simulink model "flatball_hummel_mdl_validation_IC"  (R2021b)
settings: Solver=ode1be  StartTime=0.0  StopTime=30  FixedStep=0.001  MaxStep=0.01  MinStep=0.01  RelTol=1e-3
values from neighbouring files (symbols this model uses):
  amb = evalin( 'base', 'amb')    [flatball_6dof_eqom.m]
  disc = evalin( 'base', 'disc')    [flatball_6dof_eqom.m]    (also in flatball_6dof_init.m = struct; flatball_init_disc_params.m = struct)
  k_launch_F_t_release = 0.60    (= 0.6)    [flatball_6dof_hucker_init.m]
  k_launch_Fx_kd = 2e-2    (= 0.02)    [flatball_6dof_hucker_init.m]
  k_launch_Fx_ki = 15    [flatball_6dof_hucker_init.m]
  k_launch_Fx_kp = 7.5    [flatball_6dof_hucker_init.m]
  k_launch_Fx_sat_hi = 150    [flatball_6dof_hucker_init.m]
  k_launch_Fx_sat_lo = -150    [flatball_6dof_hucker_init.m]
  k_launch_Fx_t_launch_begin = 0.50    (= 0.5)    [flatball_6dof_hucker_init.m]
  k_launch_Fx_t_launch_end = k_launch_F_t_release    (= 0.6)    [flatball_6dof_hucker_init.m]
  k_launch_Fx_tau = 1e-2    (= 0.01)    [flatball_6dof_hucker_init.m]
  k_launch_Fy_kd = k_launch_Fx_kd    (= 0.02)    [flatball_6dof_hucker_init.m]
  k_launch_Fy_ki = k_launch_Fx_ki    (= 15)    [flatball_6dof_hucker_init.m]
  k_launch_Fy_kp = k_launch_Fx_kp    (= 7.5)    [flatball_6dof_hucker_init.m]
  k_launch_Fy_sat_hi = k_launch_Fx_sat_hi    (= 150)    [flatball_6dof_hucker_init.m]
  k_launch_Fy_sat_lo = k_launch_Fx_sat_lo    (= -150)    [flatball_6dof_hucker_init.m]
  k_launch_Fy_t_launch_begin = 0.50    (= 0.5)    [flatball_6dof_hucker_init.m]
  k_launch_Fy_t_launch_end = k_launch_F_t_release    (= 0.6)    [flatball_6dof_hucker_init.m]
  k_launch_Fy_tau = 1e-2    (= 0.01)    [flatball_6dof_hucker_init.m]
  k_launch_Fz_kd = 2.5    [flatball_6dof_hucker_init.m]
  k_launch_Fz_ki = 50    [flatball_6dof_hucker_init.m]
  k_launch_Fz_kp = 20    [flatball_6dof_hucker_init.m]
  k_launch_Fz_sat_hi = 25    [flatball_6dof_hucker_init.m]
  k_launch_Fz_sat_lo = -25    [flatball_6dof_hucker_init.m]
  k_launch_Fz_t_launch_begin = 0.10    (= 0.1)    [flatball_6dof_hucker_init.m]
  k_launch_Fz_t_launch_end = k_launch_F_t_release    (= 0.6)    [flatball_6dof_hucker_init.m]
  k_launch_Fz_tau = 1e-2    (= 0.01)    [flatball_6dof_hucker_init.m]
  k_launch_M_t_release = 0.60    (= 0.6)    [flatball_6dof_hucker_init.m]
  k_launch_Mx_kd = 0.125    [flatball_6dof_hucker_init.m]
  k_launch_Mx_ki = 1.125    [flatball_6dof_hucker_init.m]
  k_launch_Mx_kp = 3.5    [flatball_6dof_hucker_init.m]
  k_launch_Mx_sat_hi = 2.5    [flatball_6dof_hucker_init.m]
  k_launch_Mx_sat_lo = -2.5    [flatball_6dof_hucker_init.m]
  k_launch_Mx_t_launch_begin = 0.30    (= 0.3)    [flatball_6dof_hucker_init.m]
  k_launch_Mx_t_launch_end = k_launch_M_t_release    (= 0.6)    [flatball_6dof_hucker_init.m]
  k_launch_Mx_tau = 1e-2    (= 0.01)    [flatball_6dof_hucker_init.m]
  k_launch_My_kd = 0.1125    [flatball_6dof_hucker_init.m]
  k_launch_My_ki = 5.5    [flatball_6dof_hucker_init.m]
  k_launch_My_kp = 4.25    [flatball_6dof_hucker_init.m]
  k_launch_My_sat_hi = 2.5    [flatball_6dof_hucker_init.m]
  k_launch_My_sat_lo = -2.5    [flatball_6dof_hucker_init.m]
  k_launch_My_t_launch_begin = 0.40    (= 0.4)    [flatball_6dof_hucker_init.m]
  k_launch_My_t_launch_end = k_launch_M_t_release    (= 0.6)    [flatball_6dof_hucker_init.m]
  k_launch_My_tau = 1e-2    (= 0.01)    [flatball_6dof_hucker_init.m]
  k_launch_Mz_kd = 1e-8    (= 1e-08)    [flatball_6dof_hucker_init.m]
  k_launch_Mz_ki = 0.2575    [flatball_6dof_hucker_init.m]
  k_launch_Mz_kp = 0.25    [flatball_6dof_hucker_init.m]
  k_launch_Mz_sat_hi = 7.5    [flatball_6dof_hucker_init.m]
  k_launch_Mz_sat_lo = -7.5    [flatball_6dof_hucker_init.m]
  k_launch_Mz_t_launch_begin = 0.20    (= 0.2)    [flatball_6dof_hucker_init.m]
  k_launch_Mz_t_launch_end = k_launch_M_t_release    (= 0.6)    [flatball_6dof_hucker_init.m]
  k_launch_Mz_tau = 1e-2    (= 0.01)    [flatball_6dof_hucker_init.m]
  X0_crowther_f2302 = [      -0.90 -0.63 -0.91,  4.48 12.52 1.84,      -0.07 0.21 5.03,    -26.25 -5.19 52.85]    [hummel_thesis_mdl_validation.m]
  X0_desired = X0_crowther_f2302    [hummel_thesis_mdl_validation.m]
  X0_hummel_f2302 = [      -0.90 -0.63 -0.91,  13.42 -0.41 0.001,      -0.07 0.21 5.03,    -14.94 -1.48 54.25]    [hummel_thesis_mdl_validation.m]
libraries: slpidlib x6, simulink x2, aerolibanim x2, aerolibnav x2, matrix_library x2, mspfiltlib x1
(part 1 of 3)
settings Model: Creator=schae  LastModifiedBy=schae
settings SolverCC: InitialStep=0.01
settings DataIOCC: SaveFormat=StructureWithTime  SaveOutput=off  DSMLogging=off  SaveTime=off  ReturnWorkspaceOutputs=off  ReturnWorkspaceOutputsName=simout

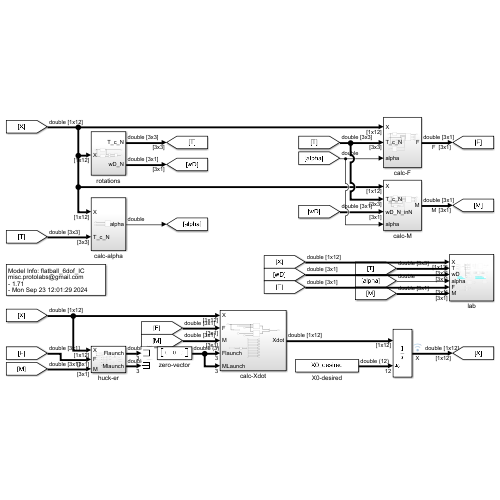
[thumbnail: Simulink's stored preview of the top-level diagram]
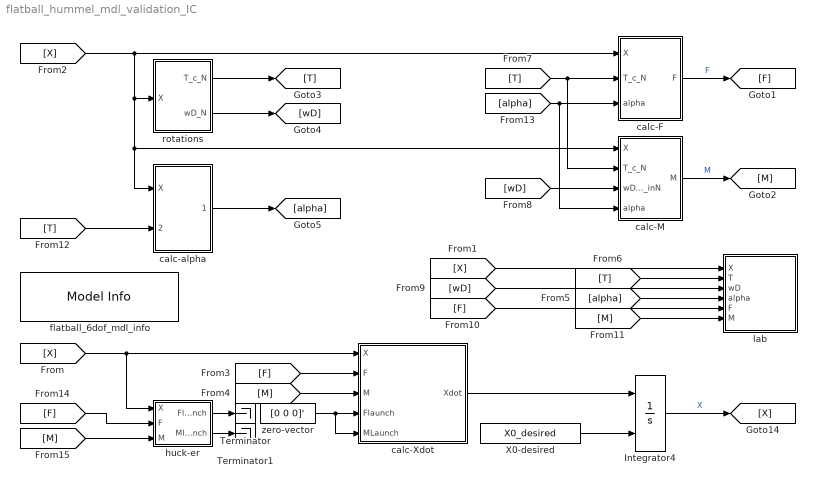
== system flatball_hummel_mdl_validation_IC ==
  Integrator4 : Integrator  InitialConditionSource=external
  Terminator : Terminator
  Terminator1 : Terminator
  X0-desired : Constant  Value=X0_desired
  calc-F : Subsystem
  calc-M : Subsystem
  calc-Xdot : Subsystem
  calc-alpha : Subsystem
  flatball_6dof_mdl_info : simulink/Model-Wide Utilities/Model Info  Frame=on  DisplayStringWithTags=|  HorizontalTextAlignment=Left  LeftAlignmentValue=0.02
      | Model Info: flatball_6dof_IC
      | misc.protolabs@gmail.com
      | - %<ModelVersion>
      | - %<LastModificationDate>
  huck-er : Subsystem
  lab : Subsystem
  rotations : Subsystem
  zero-vector : Constant  Value=[0 0 0]'
  wires:
  X0-desired/1 -> Integrator4/2
  Integrator4/1 -> [X]  "X"
  [X] -> calc-Xdot/1(X), huck-er/1(X)
  [wD] -> calc-M/3(wD_N_inN)
  rotations/1(T_c_N) -> [T]
  rotations/2(wD_N) -> [wD]
  calc-F/1(F) -> [F]  "F"
  calc-M/1(M) -> [M]  "M"
  [T] -> calc-M/2(T_c_N), calc-F/2(T_c_N)
  [X] -> calc-alpha/1(X), calc-M/1(X), rotations/1(X), calc-F/1(X)
  [X] -> lab/1(X)
  [T] -> lab/2(T)
  [wD] -> lab/3(wD)
  [F] -> lab/5(F)
  [M] -> lab/6(M)
  [alpha] -> lab/4(alpha)
  [F] -> calc-Xdot/2(F)
  [M] -> calc-Xdot/3(M)
  calc-Xdot/1(Xdot) -> Integrator4/1
  [T] -> calc-alpha/2(T_c_N)
  calc-alpha/1(alpha) -> [alpha]
  [alpha] -> calc-F/3(alpha), calc-M/4(alpha)
  [F] -> huck-er/2(F)
  [M] -> huck-er/3(M)
  huck-er/1(Flaunch) -> Terminator/1
  huck-er/2(Mlaunch) -> Terminator1/1
  zero-vector/1 -> calc-Xdot/5(MLaunch), calc-Xdot/4(Flaunch)

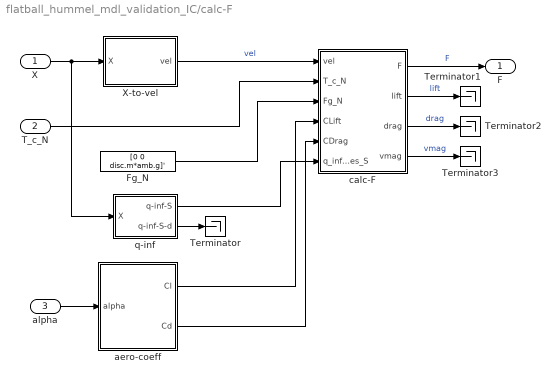
== system flatball_hummel_mdl_validation_IC/calc-F ==
  X : Inport
  T_c_N : Inport  Port=2
  alpha : Inport  Port=3
  Fg_N : Constant  Value=[0 0 disc.m*amb.g]'
  Terminator{,1..3} (4 alike) : Terminator
  X-to-vel : MATLAB Function  TreatAsAtomicUnit=on
  aero-coeff : Subsystem
  calc-F : MATLAB Function  TreatAsAtomicUnit=on
  q-inf : Subsystem
  F : Outport
  wires:
  X-to-vel/1(vel) -> calc-F/1(vel)  "vel"
  X/1 -> q-inf/1(X), X-to-vel/1(X)
  T_c_N/1 -> calc-F/2(T_c_N)
  Fg_N/1 -> calc-F/3(Fg_N)
  calc-F/1(F) -> F/1  "F"
  q-inf/1(q-inf-S) -> calc-F/6(q_inf_times_S)
  alpha/1 -> aero-coeff/1(alpha)
  aero-coeff/1(Cl) -> calc-F/4(CLift)
  aero-coeff/2(Cd) -> calc-F/5(CDrag)
  q-inf/2(q-inf-S-d) -> Terminator/1
  calc-F/2(lift) -> Terminator1/1  "lift"
  calc-F/3(drag) -> Terminator2/1  "drag"
  calc-F/4(vmag) -> Terminator3/1  "vmag"

== system flatball_hummel_mdl_validation_IC/calc-M ==
  X : Inport
  T_c_N : Inport  Port=2
  wD_N_inN : Inport  Port=3
  alpha : Inport  Port=4
  Terminator{,1..3} (4 alike) : Terminator
  X-to-vel : MATLAB Function  TreatAsAtomicUnit=on
  aero-coeff : Subsystem
  calc-M : MATLAB Function  TreatAsAtomicUnit=on
  q-inf : Subsystem
  M : Outport
  wires:
  alpha/1 -> aero-coeff/1(alpha)
  calc-M/1(M) -> M/1  "M"
  T_c_N/1 -> calc-M/2(T_c_N)
  X/1 -> X-to-vel/1(X), q-inf/1(X)
  X-to-vel/1(vel) -> calc-M/1(vel)
  q-inf/2(q-inf-S-d) -> calc-M/5(q_inf_times_Sd)
  aero-coeff/1(Cm) -> calc-M/4(CMpitch)
  wD_N_inN/1 -> calc-M/3(wD_N_inN)
  q-inf/1(q-inf-S) -> Terminator/1
  calc-M/2(p) -> Terminator1/1  "p"
  calc-M/3(q) -> Terminator2/1  "q"
  calc-M/4(r) -> Terminator3/1  "r"

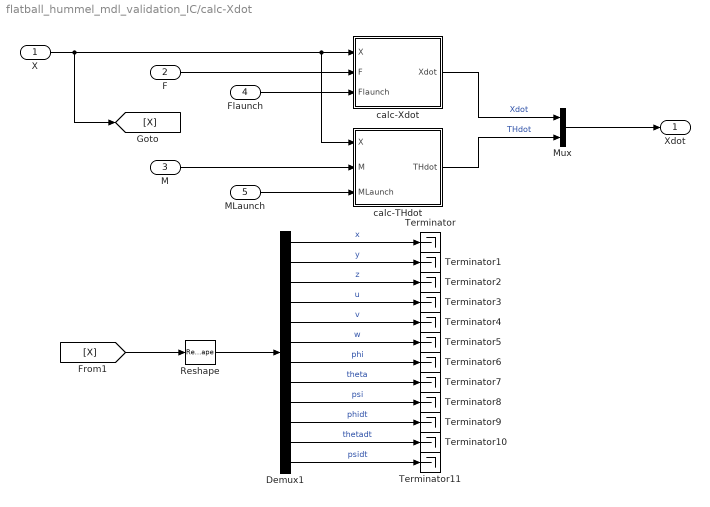
== system flatball_hummel_mdl_validation_IC/calc-Xdot ==
  X : Inport
  F : Inport  Port=2
  M : Inport  Port=3
  Flaunch : Inport  Port=4
  MLaunch : Inport  Port=5
  Demux1 : Demux  Outputs=[1 1 1 1 1 1 1 1 1 1 1 1]
  Mux : Mux  Inputs=2
  Reshape : Reshape
  Terminator{,1..11} (12 alike) : Terminator
  calc-THdot : MATLAB Function  TreatAsAtomicUnit=on
  calc-Xdot : MATLAB Function  TreatAsAtomicUnit=on
  Xdot : Outport
  wires:
  calc-Xdot/1(Xdot) -> Mux/1  "Xdot"
  Mux/1 -> Xdot/1
  X/1 -> calc-THdot/1(X), calc-Xdot/1(X), [X]
  M/1 -> calc-THdot/2(M)
  F/1 -> calc-Xdot/2(F)
  calc-THdot/1(THdot) -> Mux/2  "THdot"
  MLaunch/1 -> calc-THdot/3(MLaunch)
  Flaunch/1 -> calc-Xdot/3(Flaunch)
  Demux1/1 -> Terminator/1  "x"
  Demux1/2 -> Terminator1/1  "y"
  Demux1/3 -> Terminator2/1  "z"
  Demux1/6 -> Terminator5/1  "w"
  Demux1/5 -> Terminator4/1  "v"
  Demux1/4 -> Terminator3/1  "u"
  Demux1/10 -> Terminator9/1  "phidt"
  Demux1/11 -> Terminator10/1  "thetadt"
  Demux1/12 -> Terminator11/1  "psidt"
  Demux1/9 -> Terminator8/1  "psi"
  Demux1/8 -> Terminator7/1  "theta"
  Demux1/7 -> Terminator6/1  "phi"
  [X] -> Reshape/1
  Reshape/1 -> Demux1/1

== system flatball_hummel_mdl_validation_IC/calc-alpha ==
  X : Inport
  T_c_N : Inport  Port=2
  calc-alpha : MATLAB Function  TreatAsAtomicUnit=on
  alpha : Outport
  wires:
  calc-alpha/1(alpha) -> alpha/1  "alpha"
  X/1 -> calc-alpha/1(X)
  T_c_N/1 -> calc-alpha/2(T_c_N)

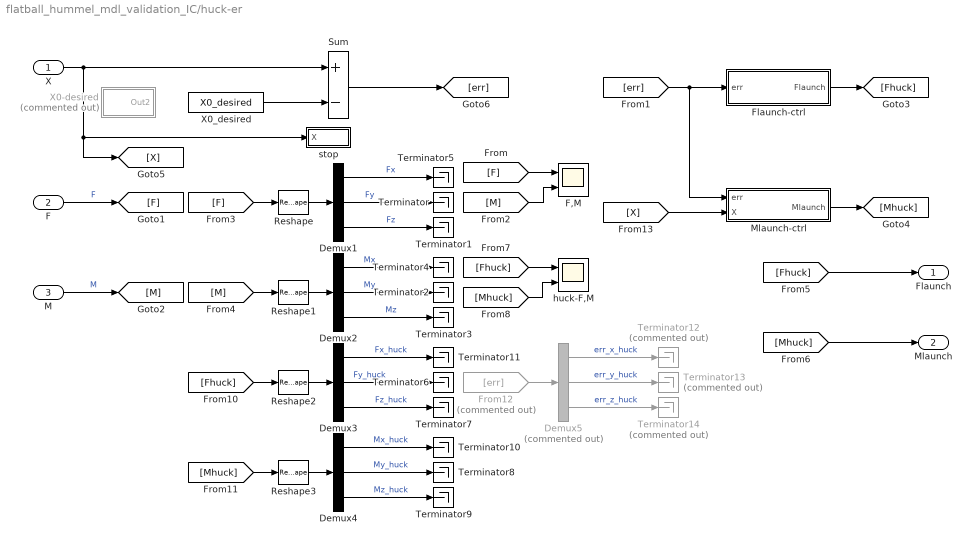
== system flatball_hummel_mdl_validation_IC/huck-er ==
  X : Inport
  F : Inport  Port=2
  M : Inport  Port=3
  Demux{1..4} (4 alike) : Demux  Outputs=3
  Demux5 : Demux  Commented=on  Outputs=3
  F,M : Scope  NumInputPorts=2
  Flaunch-ctrl : Subsystem
  From12 : From  Commented=on  GotoTag=err
  Mlaunch-ctrl : Subsystem
  Reshape{,1..3} (4 alike) : Reshape
  Sum : Sum  Inputs=+-
  Terminator{,1..11} (12 alike) : Terminator
  Terminator12 : Terminator  Commented=on
  Terminator13 : Terminator  Commented=on
  Terminator14 : Terminator  Commented=on
  X0-desired : Subsystem  Commented=on
  X0_desired : Constant  Value=X0_desired
  huck-F,M : Scope  NumInputPorts=2
  stop : Subsystem
  Flaunch : Outport
  Mlaunch : Outport  Port=2
  wires:
  X/1 -> Sum/1, [X], stop/1(X)
  Sum/1 -> [err]
  X0_desired/1 -> Sum/2
  [err] -> Mlaunch-ctrl/1(err), Flaunch-ctrl/1(err)
  F/1 -> [F]  "F"
  M/1 -> [M]  "M"
  [F] -> F,M/1
  [M] -> F,M/2
  [F] -> Reshape/1
  [M] -> Reshape1/1
  Demux1/1 -> Terminator5/1  "Fx"
  Demux1/2 -> Terminator/1  "Fy"
  Demux1/3 -> Terminator1/1  "Fz"
  Demux2/3 -> Terminator3/1  "Mz"
  Demux2/2 -> Terminator2/1  "My"
  Demux2/1 -> Terminator4/1  "Mx"
  Flaunch-ctrl/1(Flaunch) -> [Fhuck]
  Mlaunch-ctrl/1(Mlaunch) -> [Mhuck]
  [Fhuck] -> Flaunch/1
  [Mhuck] -> Mlaunch/1
  [Fhuck] -> huck-F,M/1
  [Mhuck] -> huck-F,M/2
  [X] -> Mlaunch-ctrl/2(X)
  Demux4/1 -> Terminator10/1  "Mx_huck"
  Demux4/2 -> Terminator8/1  "My_huck"
  Demux4/3 -> Terminator9/1  "Mz_huck"
  Demux3/3 -> Terminator7/1  "Fz_huck"
  Demux3/2 -> Terminator6/1  "Fy_huck"
  Demux3/1 -> Terminator11/1  "Fx_huck"
  [Mhuck] -> Reshape3/1
  [Fhuck] -> Reshape2/1
  From12/1 -> Demux5/1
  Demux5/1 -> Terminator12/1  "err_x_huck"
  Demux5/2 -> Terminator13/1  "err_y_huck"
  Demux5/3 -> Terminator14/1  "err_z_huck"
  Reshape/1 -> Demux1/1
  Reshape1/1 -> Demux2/1
  Reshape2/1 -> Demux3/1
  Reshape3/1 -> Demux4/1

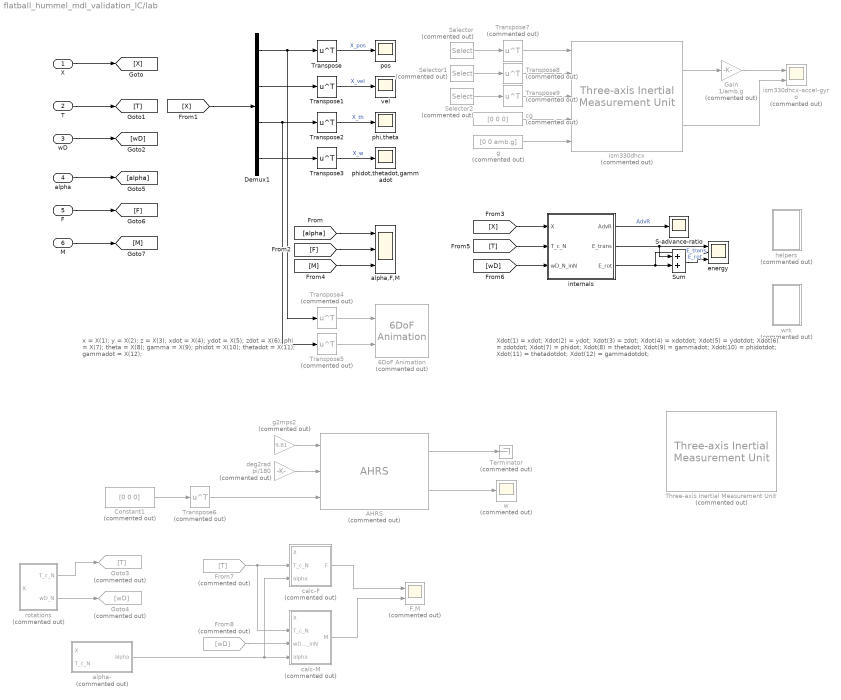
== system flatball_hummel_mdl_validation_IC/lab ==
  note: x = X(1); y = X(2); z = X(3);
      | xdot = X(4); ydot = X(5); zdot = X(6);
      |
      | phi = X(7); theta = X(8); gamma = X(9);
      | phidot = X(10); thetadot = X(11); gammadot = X(12);
  note: Xdot(1) = xdot; Xdot(2) = ydot; Xdot(3) = zdot;
      | Xdot(4) = xdotdot; Xdot(5) = ydotdot; Xdot(6) = zdotdot;
      |
      | Xdot(7) = phidot; Xdot(8) = thetadot; Xdot(9) = gammadot;
      | Xdot(10) = phidotdot; Xdot(11) = thetadotdot; Xdot(12) = gammadotdot;
  X : Inport
  T : Inport  Port=2
  wD : Inport  Port=3
  alpha : Inport  Port=4
  F : Inport  Port=5
  M : Inport  Port=6
  6DoF Animation : aerolibanim/6DoF Animation  Commented=on  u1=[-20 50 -20 50 -20 5]  u2=0.1  u3=1.0  u4=[-1 -1 -1]  u5=Fixed position  u6=[-200 -20 -10]  u7=10  u8=on
  AHRS : mspfiltlib/AHRS  Commented=on  DispRefFrame=ENU  DecimationFactor=1  InitialProcessNoise=ahrsfilter.defaultProcessNoise  OrientationFormat=Rotation matrix  SimulateUsing=Interpreted execution  AccelerometerNoise=0.0001924722  GyroscopeNoise=9.1385e-5  MagnetometerNoise=0.1  GyroscopeDriftNoise=3.0462e-13  LinearAccelerationNoise=0.0096236100000000012  MagneticDisturbanceNoise=0.5  LinearAccelerationDecayFactor=0.5  MagneticDisturbanceDecayFactor=0.5  ExpectedMagneticFieldStrength=50
      settings: SourceProductBaseCode=TF,NV
  Constant1 : Constant  Commented=on  Value=[0 0 0]
  Demux1 : Demux  Outputs=[3 3 3 3]
  F,M : Scope  Commented=on  NumInputPorts=2
  From7 : From  Commented=on  GotoTag=T
  From8 : From  Commented=on  GotoTag=wD
  Gain : Gain  Commented=on  Gain=1/amb.g
  Goto3 : Goto  Commented=on  GotoTag=T
  Goto4 : Goto  Commented=on  GotoTag=wD
  S-advance-ratio : Scope
  Selector : Selector  Commented=on  InputPortWidth=12  IndexOptions=Index vector (dialog)  Indices=[4 5 6]  OutputSizes=1
  Selector1 : Selector  Commented=on  InputPortWidth=12  IndexOptions=Index vector (dialog)  Indices=[7 8 9]  OutputSizes=1
  Selector2 : Selector  Commented=on  InputPortWidth=12  IndexOptions=Index vector (dialog)  Indices=[7 8 9]  OutputSizes=1
  Sum : Sum  Inputs=2
  Terminator : Terminator  Commented=on
  Three-axis Inertial Measurement Unit : aerolibnav/Three-axis Inertial Measurement Unit  Commented=on  units=Metric (MKS)  imu=[0 0 0]  i_Ts=0  dtype_a=on  w_a=190  z_a=0.707  a_sf_cc=[1 0 0; 0 1 0; 0 0 1]  a_bias=[0 0 0]  a_sat="[-inf  -inf  -inf  inf inf inf]"  dtype_g=on  w_g=190  z_g=0.707  g_sf_cc=[1 0 0; 0 1 0; 0 0 1]  g_bias=[0 0 0]  g_sens=[0 0 0]  g_sat="[-inf  -inf  -inf  inf inf inf]"  i_rand=on  i_seeds=[23093 23094 23095 23096 23097 23098]  i_pow=[0.001 0.001 0.001 0.0001 0.0001 0.0001]
  Transpose{,1..3} (4 alike) : Math  Operator=transpose  SaturateOnIntegerOverflow=on
  Transpose{4..9} (6 alike) : Math  Commented=on  Operator=transpose  SaturateOnIntegerOverflow=on
  alpha,F,M : Scope  NumInputPorts=3
  alpha- : MATLAB Function  Commented=on  TreatAsAtomicUnit=on
  calc-F : Subsystem  Commented=on
  calc-M : Subsystem  Commented=on
  cg : Constant  Commented=on  Value=[0 0 0]
  deg2rad : Gain  Commented=on  Gain=pi/180
  energy : Scope  NumInputPorts=3
  g : Constant  Commented=on  Value=[0 0 amb.g]
  g2mps2 : Gain  Commented=on  Gain=9.81
  helpers : Subsystem  Commented=on
  internals : MATLAB Function  TreatAsAtomicUnit=on
  ism330dhcx : aerolibnav/Three-axis Inertial Measurement Unit  Commented=on  units=Metric (MKS)  imu=[-2e-3 1e-3 -5e-3]  i_Ts=0  dtype_a=on  w_a=190  z_a=0.707  a_sf_cc=[1 0 0; 0 1 0; 0 0 1]  a_bias=[0 0 0]  a_sat="[-inf  -inf  -inf  inf inf inf]"  dtype_g=on  w_g=190  z_g=0.707  g_sf_cc=[1 0 0; 0 1 0; 0 0 1]  g_bias=[0 0 0]  g_sens=[0 0 0]  g_sat="[-inf  -inf  -inf  inf inf inf]"  i_rand=on  i_seeds=[23093 23094 23095 23096 23097 23098]  i_pow=[0.001 0.001 0.001 0.0001 0.0001 0.0001]
  ism330dhcx-accel-gyro : Scope  Commented=on  NumInputPorts=2
  phi,theta : Scope
  phidot,thetadot,gammadot : Scope
  pos : Scope
  rotations : Subsystem  Commented=on
  vel : Scope
  w : Scope  Commented=on
  wrk : Subsystem  Commented=on
  wires:
  From7/1 -> calc-M/2(T_c_N), calc-F/2(T_c_N)
  alpha-/1(alpha) -> calc-F/3(alpha), calc-M/4(alpha)
  From8/1 -> calc-M/3(wD_N_inN)
  calc-M/1(M) -> F,M/2
  calc-F/1(F) -> F,M/1
  rotations/1(T_c_N) -> Goto3/1
  rotations/2(wD_N) -> Goto4/1
  internals/3(E_rot) -> Sum/2, energy/2  "E_rot"
  [wD] -> internals/3(wD_N_inN)
  internals/1(AdvR) -> S-advance-ratio/1  "AdvR"
  [T] -> internals/2(T_c_N)
  Sum/1 -> energy/3
  [X] -> internals/1(X)
  internals/2(E_trans) -> Sum/1, energy/1  "E_trans"
  Demux1/4 -> Transpose3/1
  Demux1/3 -> Transpose5/1, Transpose2/1
  Demux1/1 -> Transpose4/1, Transpose/1
  Demux1/2 -> Transpose1/1
  [X] -> Demux1/1
  X/1 -> [X]
  T/1 -> [T]
  wD/1 -> [wD]
  F/1 -> [F]
  alpha/1 -> [alpha]
  M/1 -> [M]
  [alpha] -> alpha,F,M/1
  [F] -> alpha,F,M/2
  [M] -> alpha,F,M/3
  Transpose/1 -> pos/1  "X_pos"
  Transpose1/1 -> vel/1  "X_vel"
  Transpose2/1 -> phi,theta/1  "X_th"
  Transpose3/1 -> phidot,thetadot,gammadot/1  "X_w"
  Transpose4/1 -> 6DoF Animation/1
  Transpose5/1 -> 6DoF Animation/2
  Transpose6/1 -> AHRS/3
  Constant1/1 -> Transpose6/1
  AHRS/2 -> w/1
  g2mps2/1 -> AHRS/1
  deg2rad/1 -> AHRS/2
  AHRS/1 -> Terminator/1
  Transpose7/1 -> ism330dhcx/1
  Selector/1 -> Transpose7/1
  g/1 -> ism330dhcx/5
  Transpose8/1 -> ism330dhcx/2
  cg/1 -> ism330dhcx/4
  ism330dhcx/1 -> Gain/1
  Transpose9/1 -> ism330dhcx/3
  Selector1/1 -> Transpose8/1
  Selector2/1 -> Transpose9/1
  Gain/1 -> ism330dhcx-accel-gyro/1
  ism330dhcx/2 -> ism330dhcx-accel-gyro/2

== system flatball_hummel_mdl_validation_IC/rotations ==
  X : Inport
  MatrixMultiply3 : Product  Multiplication=Matrix(*)
  Transpose : Math  Operator=transpose  SaturateOnIntegerOverflow=on
  Transpose1 : Math  Operator=transpose  SaturateOnIntegerOverflow=on
  X-to-T_c_N : MATLAB Function  TreatAsAtomicUnit=on
  X-to-wD_N_inC : MATLAB Function  TreatAsAtomicUnit=on
  T_c_N : Outport
  wD_N : Outport  Port=2
  wires:
  X-to-T_c_N/1(T_c_N) -> Transpose1/1, T_c_N/1
  Transpose1/1 -> MatrixMultiply3/1
  X-to-wD_N_inC/1(wD_N_inC) -> Transpose/1
  Transpose/1 -> MatrixMultiply3/2
  MatrixMultiply3/1 -> wD_N/1
  X/1 -> X-to-wD_N_inC/1(X), X-to-T_c_N/1(X)

== system flatball_hummel_mdl_validation_IC/calc-F/aero-coeff ==
  alpha : Inport
  calc-Cd : Subsystem
  calc-Cl : Subsystem
  Cl : Outport
  Cd : Outport  Port=2
  wires:
  alpha/1 -> calc-Cl/1(alpha), calc-Cd/1(alpha)
  calc-Cl/1(Cl) -> Cl/1  "Cl"
  calc-Cd/1(Cd) -> Cd/1  "Cd"

== system flatball_hummel_mdl_validation_IC/calc-F/q-inf ==
  X : Inport
  Gain : Gain  Gain=0.5
  Product1 : Product  Inputs=3
  Product2 : Product
  S : Constant  Value=disc.A
  Square : Math  Operator=square  SaturateOnIntegerOverflow=on
  X-to-vel : MATLAB Function  TreatAsAtomicUnit=on
  d : Constant  Value=disc.d
  rho : Constant  Value=amb.rho
  vector-norm : MATLAB Function  TreatAsAtomicUnit=on
  q-inf-S : Outport
  q-inf-S-d : Outport  Port=2
  wires:
  Product1/1 -> Gain/1
  rho/1 -> Product1/3
  X/1 -> X-to-vel/1(X)
  vector-norm/1(norm) -> Square/1
  S/1 -> Product1/2
  Square/1 -> Product1/1
  Gain/1 -> Product2/1, q-inf-S/1
  X-to-vel/1(vel) -> vector-norm/1(vec)
  Product2/1 -> q-inf-S-d/1
  d/1 -> Product2/2

== system flatball_hummel_mdl_validation_IC/calc-M/aero-coeff ==
  alpha : Inport
  Subsystem2 : Subsystem
  Cm : Outport
  wires:
  alpha/1 -> Subsystem2/1(alpha)
  Subsystem2/1(Cm) -> Cm/1  "Cm"

== system flatball_hummel_mdl_validation_IC/calc-M/q-inf ==
  X : Inport
  Gain : Gain  Gain=0.5
  Product1 : Product  Inputs=3
  Product2 : Product
  S : Constant  Value=disc.A
  Square : Math  Operator=square  SaturateOnIntegerOverflow=on
  X-to-vel : MATLAB Function  TreatAsAtomicUnit=on
  d : Constant  Value=disc.d
  rho : Constant  Value=amb.rho
  vector-norm : MATLAB Function  TreatAsAtomicUnit=on
  q-inf-S : Outport
  q-inf-S-d : Outport  Port=2
  wires:
  d/1 -> Product2/2
  Product2/1 -> q-inf-S-d/1
  X-to-vel/1(vel) -> vector-norm/1(vec)
  Gain/1 -> q-inf-S/1, Product2/1
  Square/1 -> Product1/1
  S/1 -> Product1/2
  vector-norm/1(norm) -> Square/1
  X/1 -> X-to-vel/1(X)
  rho/1 -> Product1/3
  Product1/1 -> Gain/1

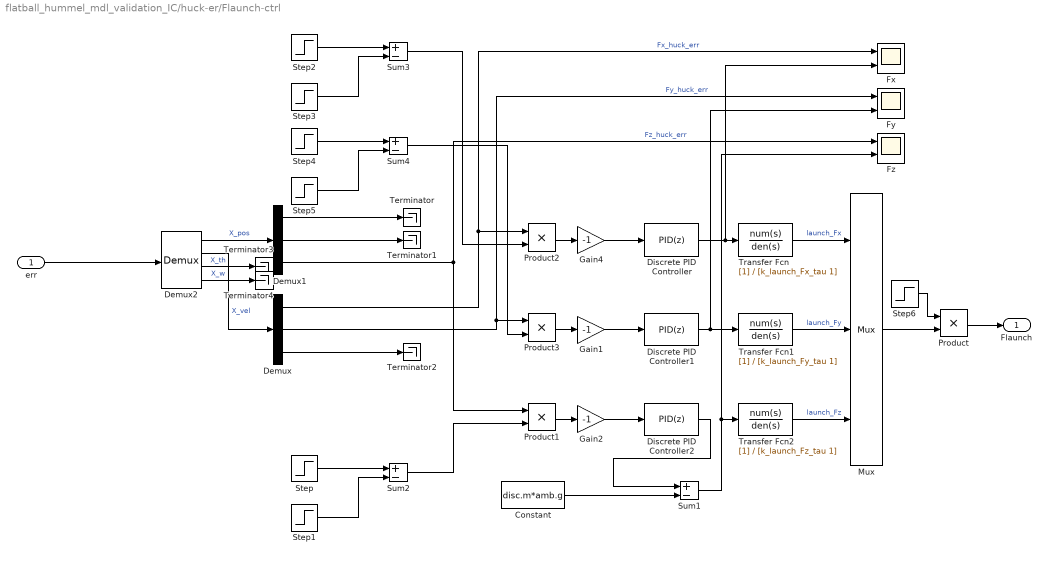
== system flatball_hummel_mdl_validation_IC/huck-er/Flaunch-ctrl ==
  err : Inport
  Constant : Constant  Value=disc.m*amb.g
  Demux : Demux  Outputs=3
  Demux1 : Demux  Outputs=3
  Demux2 : Demux  Outputs=[3 3 3 3]
  Discrete PID Controller : slpidlib/PID Controller  Controller=PID  Form=Parallel  TimeDomain=Discrete-time  UseExternalTs=off  SampleTime=-1  IntegratorMethod=Forward Euler  FilterMethod=Forward Euler  ControllerParametersSource=internal  P=k_launch_Fx_kp  I=k_launch_Fx_ki  D=k_launch_Fx_kd  UseFilter=on  N=100  TunerSelectOption=Transfer Function Based (PID Tuner App)  InitialConditionSource=internal  InitialConditionForIntegrator=0  InitialConditionForFilter=0  DifferentiatorICPrevScaledInput=0  ExternalReset=none  TrackingMode=off  Kt=1  LimitOutput=on  SatLimitsSource=internal  UpperSaturationLimit=k_launch_Fx_sat_hi  LowerSaturationLimit=k_launch_Fx_sat_lo  LinearizeAsGain=off  AntiWindupMode=clamping  Kb=1  POutMin=[]  POutMax=[]  IOutMin=[]  IOutMax=[]  DOutMin=[]  DOutMax=[]  NOutMin=[]  NOutMax=[]  SumOutMin=[]  SumOutMax=[]  SaturationOutMin=[]  SaturationOutMax=[]  PParamMin=[]  PParamMax=[]  IParamMin=[]  IParamMax=[]  DParamMin=[]  DParamMax=[]  NParamMin=[]  NParamMax=[]  KbParamMin=[]  KbParamMax=[]  KtParamMin=[]  KtParamMax=[]  KbOutMin=[]  KbOutMax=[]  KtOutMin=[]  KtOutMax=[]  IntegratorOutMin=[]  IntegratorOutMax=[]  FilterOutMin=[]  FilterOutMax=[]  SumI1OutMin=[]  SumI1OutMax=[]  SumI2OutMin=[]  SumI2OutMax=[]  SumI3OutMin=[]  SumI3OutMax=[]  SumI4OutMin=[]  SumI4OutMax=[]  SumDOutMin=[]  SumDOutMax=[]  DifferentiatorOutMin=[]  DifferentiatorOutMax=[]  FilterDiffOutCoefMin=[]  FilterDiffOutCoefMax=[]  ReciprocalOutMin=[]  ReciprocalOutMax=[]  SumDenOutMin=[]  SumDenOutMax=[]  SumNumOutMin=[]  SumNumOutMax=[]  DivideOutMin=[]  DivideOutMax=[]  UdiffTsProdOutMin=[]  UdiffTsProdOutMax=[]  NTsProdOutMin=[]  NTsProdOutMax=[]  UintegralTsProdOutMin=[]  UintegralTsProdOutMax=[]  UngainTsProdOutMin=[]  UngainTsProdOutMax=[]  IntegratorContinuousStateAttributes=''  IntegratorStateMustResolveToSignalObject=off  IntegratorRTWStateStorageClass=Auto  FilterContinuousStateAttributes=''  FilterStateMustResolveToSignalObject=off  FilterRTWStateStorageClass=Auto  ParallelPVariant=InternalParameters  IdealPVariant=Disabled  IVariant=InternalParameters  DVariant=InternalParameters  IntegratorVariant=Discrete  SatVariant=Enabled  AWVariant=DiscClampingParallel  PCopyVariant=Disabled  TRVariant=Disabled  FdbkBlocksVariant=Forward  IdealPFdbkVariant=Disabled  SatFdbkVariant=Disabled  DerivativeFilterVariant=ForwardEulerFilter  NVariant=InternalParameters  NCopyVariant=Disabled  FilterICVariant=InternalICsFilter  IntegratorICVariant=InternalICs  ExternalResetVariant=Disabled  TRSumVariant=Passthrough  SumFdbkVariant=Disabled  SumVariant=Sum_PID  TsampFilterVariant=InternalTs  TsampNgainVariant=Passthrough  TsampIntegralVariant=Passthrough  ExternalSaturationOutDataTypeStr=Inherit: Same as second input
  Discrete PID Controller1 : slpidlib/PID Controller  Controller=PID  Form=Parallel  TimeDomain=Discrete-time  UseExternalTs=off  SampleTime=-1  IntegratorMethod=Forward Euler  FilterMethod=Forward Euler  ControllerParametersSource=internal  P=k_launch_Fy_kp  I=k_launch_Fy_ki  D=k_launch_Fy_kd  UseFilter=on  N=100  TunerSelectOption=Transfer Function Based (PID Tuner App)  InitialConditionSource=internal  InitialConditionForIntegrator=0  InitialConditionForFilter=0  DifferentiatorICPrevScaledInput=0  ExternalReset=none  TrackingMode=off  Kt=1  LimitOutput=on  SatLimitsSource=internal  UpperSaturationLimit=k_launch_Fy_sat_hi  LowerSaturationLimit=k_launch_Fy_sat_lo  LinearizeAsGain=off  AntiWindupMode=clamping  Kb=1  POutMin=[]  POutMax=[]  IOutMin=[]  IOutMax=[]  DOutMin=[]  DOutMax=[]  NOutMin=[]  NOutMax=[]  SumOutMin=[]  SumOutMax=[]  SaturationOutMin=[]  SaturationOutMax=[]  PParamMin=[]  PParamMax=[]  IParamMin=[]  IParamMax=[]  DParamMin=[]  DParamMax=[]  NParamMin=[]  NParamMax=[]  KbParamMin=[]  KbParamMax=[]  KtParamMin=[]  KtParamMax=[]  KbOutMin=[]  KbOutMax=[]  KtOutMin=[]  KtOutMax=[]  IntegratorOutMin=[]  IntegratorOutMax=[]  FilterOutMin=[]  FilterOutMax=[]  SumI1OutMin=[]  SumI1OutMax=[]  SumI2OutMin=[]  SumI2OutMax=[]  SumI3OutMin=[]  SumI3OutMax=[]  SumI4OutMin=[]  SumI4OutMax=[]  SumDOutMin=[]  SumDOutMax=[]  DifferentiatorOutMin=[]  DifferentiatorOutMax=[]  FilterDiffOutCoefMin=[]  FilterDiffOutCoefMax=[]  ReciprocalOutMin=[]  ReciprocalOutMax=[]  SumDenOutMin=[]  SumDenOutMax=[]  SumNumOutMin=[]  SumNumOutMax=[]  DivideOutMin=[]  DivideOutMax=[]  UdiffTsProdOutMin=[]  UdiffTsProdOutMax=[]  NTsProdOutMin=[]  NTsProdOutMax=[]  UintegralTsProdOutMin=[]  UintegralTsProdOutMax=[]  UngainTsProdOutMin=[]  UngainTsProdOutMax=[]  IntegratorContinuousStateAttributes=''  IntegratorStateMustResolveToSignalObject=off  IntegratorRTWStateStorageClass=Auto  FilterContinuousStateAttributes=''  FilterStateMustResolveToSignalObject=off  FilterRTWStateStorageClass=Auto  ParallelPVariant=InternalParameters  IdealPVariant=Disabled  IVariant=InternalParameters  DVariant=InternalParameters  IntegratorVariant=Discrete  SatVariant=Enabled  AWVariant=DiscClampingParallel  PCopyVariant=Disabled  TRVariant=Disabled  FdbkBlocksVariant=Forward  IdealPFdbkVariant=Disabled  SatFdbkVariant=Disabled  DerivativeFilterVariant=ForwardEulerFilter  NVariant=InternalParameters  NCopyVariant=Disabled  FilterICVariant=InternalICsFilter  IntegratorICVariant=InternalICs  ExternalResetVariant=Disabled  TRSumVariant=Passthrough  SumFdbkVariant=Disabled  SumVariant=Sum_PID  TsampFilterVariant=InternalTs  TsampNgainVariant=Passthrough  TsampIntegralVariant=Passthrough  ExternalSaturationOutDataTypeStr=Inherit: Same as second input
  Discrete PID Controller2 : slpidlib/PID Controller  Controller=PID  Form=Parallel  TimeDomain=Discrete-time  UseExternalTs=off  SampleTime=-1  IntegratorMethod=Forward Euler  FilterMethod=Forward Euler  ControllerParametersSource=internal  P=k_launch_Fz_kp  I=k_launch_Fz_ki  D=k_launch_Fz_kd  UseFilter=on  N=100  TunerSelectOption=Transfer Function Based (PID Tuner App)  InitialConditionSource=internal  InitialConditionForIntegrator=0  InitialConditionForFilter=0  DifferentiatorICPrevScaledInput=0  ExternalReset=none  TrackingMode=off  Kt=1  LimitOutput=on  SatLimitsSource=internal  UpperSaturationLimit=k_launch_Fz_sat_hi  LowerSaturationLimit=k_launch_Fz_sat_lo  LinearizeAsGain=off  AntiWindupMode=clamping  Kb=1  POutMin=[]  POutMax=[]  IOutMin=[]  IOutMax=[]  DOutMin=[]  DOutMax=[]  NOutMin=[]  NOutMax=[]  SumOutMin=[]  SumOutMax=[]  SaturationOutMin=[]  SaturationOutMax=[]  PParamMin=[]  PParamMax=[]  IParamMin=[]  IParamMax=[]  DParamMin=[]  DParamMax=[]  NParamMin=[]  NParamMax=[]  KbParamMin=[]  KbParamMax=[]  KtParamMin=[]  KtParamMax=[]  KbOutMin=[]  KbOutMax=[]  KtOutMin=[]  KtOutMax=[]  IntegratorOutMin=[]  IntegratorOutMax=[]  FilterOutMin=[]  FilterOutMax=[]  SumI1OutMin=[]  SumI1OutMax=[]  SumI2OutMin=[]  SumI2OutMax=[]  SumI3OutMin=[]  SumI3OutMax=[]  SumI4OutMin=[]  SumI4OutMax=[]  SumDOutMin=[]  SumDOutMax=[]  DifferentiatorOutMin=[]  DifferentiatorOutMax=[]  FilterDiffOutCoefMin=[]  FilterDiffOutCoefMax=[]  ReciprocalOutMin=[]  ReciprocalOutMax=[]  SumDenOutMin=[]  SumDenOutMax=[]  SumNumOutMin=[]  SumNumOutMax=[]  DivideOutMin=[]  DivideOutMax=[]  UdiffTsProdOutMin=[]  UdiffTsProdOutMax=[]  NTsProdOutMin=[]  NTsProdOutMax=[]  UintegralTsProdOutMin=[]  UintegralTsProdOutMax=[]  UngainTsProdOutMin=[]  UngainTsProdOutMax=[]  IntegratorContinuousStateAttributes=''  IntegratorStateMustResolveToSignalObject=off  IntegratorRTWStateStorageClass=Auto  FilterContinuousStateAttributes=''  FilterStateMustResolveToSignalObject=off  FilterRTWStateStorageClass=Auto  ParallelPVariant=InternalParameters  IdealPVariant=Disabled  IVariant=InternalParameters  DVariant=InternalParameters  IntegratorVariant=Discrete  SatVariant=Enabled  AWVariant=DiscClampingParallel  PCopyVariant=Disabled  TRVariant=Disabled  FdbkBlocksVariant=Forward  IdealPFdbkVariant=Disabled  SatFdbkVariant=Disabled  DerivativeFilterVariant=ForwardEulerFilter  NVariant=InternalParameters  NCopyVariant=Disabled  FilterICVariant=InternalICsFilter  IntegratorICVariant=InternalICs  ExternalResetVariant=Disabled  TRSumVariant=Passthrough  SumFdbkVariant=Disabled  SumVariant=Sum_PID  TsampFilterVariant=InternalTs  TsampNgainVariant=Passthrough  TsampIntegralVariant=Passthrough  ExternalSaturationOutDataTypeStr=Inherit: Same as second input
  Fx : Scope  NumInputPorts=2
  Fy : Scope  NumInputPorts=2
  Fz : Scope  NumInputPorts=2
  Gain1 : Gain  Gain=-1
  Gain2 : Gain  Gain=-1
  Gain4 : Gain  Gain=-1
  Mux : Mux  Inputs=3
  Product{,1..3} (4 alike) : Product
  Step : Step  Time=k_launch_Fz_t_launch_begin  SampleTime=0
  Step1 : Step  Time=k_launch_Fz_t_launch_end  SampleTime=0
  Step2 : Step  Time=k_launch_Fx_t_launch_begin  SampleTime=0
  Step3 : Step  Time=k_launch_Fx_t_launch_end  SampleTime=0
  Step4 : Step  Time=k_launch_Fy_t_launch_begin  SampleTime=0
  Step5 : Step  Time=k_launch_Fy_t_launch_end  SampleTime=0
  Step6 : Step  Time=k_launch_F_t_release  Before=1  After=0  SampleTime=0
  Sum{1..4} (4 alike) : Sum  Inputs=+-
  Terminator{,1..4} (5 alike) : Terminator
  Transfer Fcn : TransferFcn  Denominator=[k_launch_Fx_tau 1]
  Transfer Fcn1 : TransferFcn  Denominator=[k_launch_Fy_tau 1]
  Transfer Fcn2 : TransferFcn  Denominator=[k_launch_Fz_tau 1]
  Flaunch : Outport
  wires:
  Gain1/1 -> Discrete PID Controller1/1
  Transfer Fcn/1 -> Mux/1  "launch_Fx"
  Transfer Fcn1/1 -> Mux/2  "launch_Fy"
  Transfer Fcn2/1 -> Mux/3  "launch_Fz"
  Step6/1 -> Product/1
  Mux/1 -> Product/2
  Product/1 -> Flaunch/1
  Demux/1 -> Product2/1, Fx/1  "Fx_huck_err"
  Gain4/1 -> Discrete PID Controller/1
  Discrete PID Controller/1 -> Fx/2, Transfer Fcn/1
  Discrete PID Controller1/1 -> Fy/2, Transfer Fcn1/1
  Demux/2 -> Product3/1, Fy/1  "Fy_huck_err"
  Discrete PID Controller2/1 -> Sum1/1
  Constant/1 -> Sum1/2
  Sum1/1 -> Fz/2, Transfer Fcn2/1
  Gain2/1 -> Discrete PID Controller2/1
  Demux1/1 -> Terminator/1
  Demux1/2 -> Terminator1/1
  Demux/3 -> Terminator2/1
  Demux1/3 -> Product1/1, Fz/1  "Fz_huck_err"
  Step1/1 -> Sum2/2
  Step/1 -> Sum2/1
  Product1/1 -> Gain2/1
  Sum2/1 -> Product1/2
  Product3/1 -> Gain1/1
  Product2/1 -> Gain4/1
  Step2/1 -> Sum3/1
  Step3/1 -> Sum3/2
  Sum3/1 -> Product2/2
  Step5/1 -> Sum4/2
  Step4/1 -> Sum4/1
  Sum4/1 -> Product3/2
  Demux2/4 -> Terminator4/1  "X_w"
  Demux2/3 -> Terminator3/1  "X_th"
  err/1 -> Demux2/1
  Demux2/1 -> Demux1/1  "X_pos"
  Demux2/2 -> Demux/1  "X_vel"

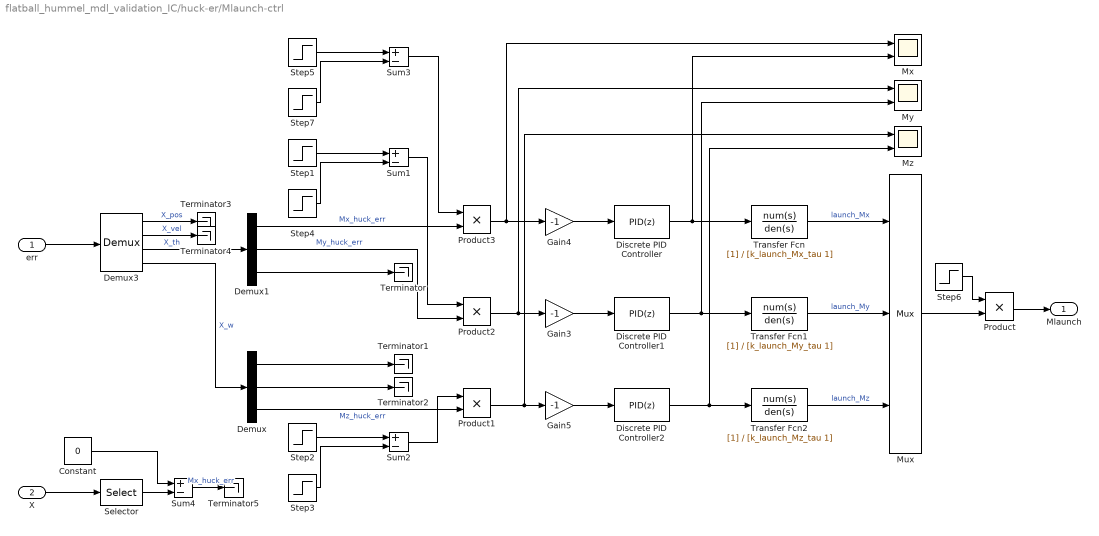
== system flatball_hummel_mdl_validation_IC/huck-er/Mlaunch-ctrl ==
  err : Inport
  X : Inport  Port=2
  Constant : Constant  Value=0
  Demux : Demux  Outputs=3
  Demux1 : Demux  Outputs=3
  Demux3 : Demux  Outputs=[3 3 3 3]
  Discrete PID Controller : slpidlib/PID Controller  Controller=PID  Form=Parallel  TimeDomain=Discrete-time  UseExternalTs=off  SampleTime=-1  IntegratorMethod=Forward Euler  FilterMethod=Forward Euler  ControllerParametersSource=internal  P=k_launch_Mx_kp  I=k_launch_Mx_ki  D=k_launch_Mx_kd  UseFilter=on  N=100  TunerSelectOption=Transfer Function Based (PID Tuner App)  InitialConditionSource=internal  InitialConditionForIntegrator=0  InitialConditionForFilter=0  DifferentiatorICPrevScaledInput=0  ExternalReset=none  TrackingMode=off  Kt=1  LimitOutput=on  SatLimitsSource=internal  UpperSaturationLimit=k_launch_Mx_sat_hi  LowerSaturationLimit=k_launch_Mx_sat_lo  LinearizeAsGain=off  AntiWindupMode=clamping  Kb=1  POutMin=[]  POutMax=[]  IOutMin=[]  IOutMax=[]  DOutMin=[]  DOutMax=[]  NOutMin=[]  NOutMax=[]  SumOutMin=[]  SumOutMax=[]  SaturationOutMin=[]  SaturationOutMax=[]  PParamMin=[]  PParamMax=[]  IParamMin=[]  IParamMax=[]  DParamMin=[]  DParamMax=[]  NParamMin=[]  NParamMax=[]  KbParamMin=[]  KbParamMax=[]  KtParamMin=[]  KtParamMax=[]  KbOutMin=[]  KbOutMax=[]  KtOutMin=[]  KtOutMax=[]  IntegratorOutMin=[]  IntegratorOutMax=[]  FilterOutMin=[]  FilterOutMax=[]  SumI1OutMin=[]  SumI1OutMax=[]  SumI2OutMin=[]  SumI2OutMax=[]  SumI3OutMin=[]  SumI3OutMax=[]  SumI4OutMin=[]  SumI4OutMax=[]  SumDOutMin=[]  SumDOutMax=[]  DifferentiatorOutMin=[]  DifferentiatorOutMax=[]  FilterDiffOutCoefMin=[]  FilterDiffOutCoefMax=[]  ReciprocalOutMin=[]  ReciprocalOutMax=[]  SumDenOutMin=[]  SumDenOutMax=[]  SumNumOutMin=[]  SumNumOutMax=[]  DivideOutMin=[]  DivideOutMax=[]  UdiffTsProdOutMin=[]  UdiffTsProdOutMax=[]  NTsProdOutMin=[]  NTsProdOutMax=[]  UintegralTsProdOutMin=[]  UintegralTsProdOutMax=[]  UngainTsProdOutMin=[]  UngainTsProdOutMax=[]  IntegratorContinuousStateAttributes=''  IntegratorStateMustResolveToSignalObject=off  IntegratorRTWStateStorageClass=Auto  FilterContinuousStateAttributes=''  FilterStateMustResolveToSignalObject=off  FilterRTWStateStorageClass=Auto  ParallelPVariant=InternalParameters  IdealPVariant=Disabled  IVariant=InternalParameters  DVariant=InternalParameters  IntegratorVariant=Discrete  SatVariant=Enabled  AWVariant=DiscClampingParallel  PCopyVariant=Disabled  TRVariant=Disabled  FdbkBlocksVariant=Forward  IdealPFdbkVariant=Disabled  SatFdbkVariant=Disabled  DerivativeFilterVariant=ForwardEulerFilter  NVariant=InternalParameters  NCopyVariant=Disabled  FilterICVariant=InternalICsFilter  IntegratorICVariant=InternalICs  ExternalResetVariant=Disabled  TRSumVariant=Passthrough  SumFdbkVariant=Disabled  SumVariant=Sum_PID  TsampFilterVariant=InternalTs  TsampNgainVariant=Passthrough  TsampIntegralVariant=Passthrough  ExternalSaturationOutDataTypeStr=Inherit: Same as second input
  Discrete PID Controller1 : slpidlib/PID Controller  Controller=PID  Form=Parallel  TimeDomain=Discrete-time  UseExternalTs=off  SampleTime=-1  IntegratorMethod=Forward Euler  FilterMethod=Forward Euler  ControllerParametersSource=internal  P=k_launch_My_kp  I=k_launch_My_ki  D=k_launch_My_kd  UseFilter=on  N=100  TunerSelectOption=Transfer Function Based (PID Tuner App)  InitialConditionSource=internal  InitialConditionForIntegrator=0  InitialConditionForFilter=0  DifferentiatorICPrevScaledInput=0  ExternalReset=none  TrackingMode=off  Kt=1  LimitOutput=on  SatLimitsSource=internal  UpperSaturationLimit=k_launch_My_sat_hi  LowerSaturationLimit=k_launch_My_sat_lo  LinearizeAsGain=off  AntiWindupMode=clamping  Kb=1  POutMin=[]  POutMax=[]  IOutMin=[]  IOutMax=[]  DOutMin=[]  DOutMax=[]  NOutMin=[]  NOutMax=[]  SumOutMin=[]  SumOutMax=[]  SaturationOutMin=[]  SaturationOutMax=[]  PParamMin=[]  PParamMax=[]  IParamMin=[]  IParamMax=[]  DParamMin=[]  DParamMax=[]  NParamMin=[]  NParamMax=[]  KbParamMin=[]  KbParamMax=[]  KtParamMin=[]  KtParamMax=[]  KbOutMin=[]  KbOutMax=[]  KtOutMin=[]  KtOutMax=[]  IntegratorOutMin=[]  IntegratorOutMax=[]  FilterOutMin=[]  FilterOutMax=[]  SumI1OutMin=[]  SumI1OutMax=[]  SumI2OutMin=[]  SumI2OutMax=[]  SumI3OutMin=[]  SumI3OutMax=[]  SumI4OutMin=[]  SumI4OutMax=[]  SumDOutMin=[]  SumDOutMax=[]  DifferentiatorOutMin=[]  DifferentiatorOutMax=[]  FilterDiffOutCoefMin=[]  FilterDiffOutCoefMax=[]  ReciprocalOutMin=[]  ReciprocalOutMax=[]  SumDenOutMin=[]  SumDenOutMax=[]  SumNumOutMin=[]  SumNumOutMax=[]  DivideOutMin=[]  DivideOutMax=[]  UdiffTsProdOutMin=[]  UdiffTsProdOutMax=[]  NTsProdOutMin=[]  NTsProdOutMax=[]  UintegralTsProdOutMin=[]  UintegralTsProdOutMax=[]  UngainTsProdOutMin=[]  UngainTsProdOutMax=[]  IntegratorContinuousStateAttributes=''  IntegratorStateMustResolveToSignalObject=off  IntegratorRTWStateStorageClass=Auto  FilterContinuousStateAttributes=''  FilterStateMustResolveToSignalObject=off  FilterRTWStateStorageClass=Auto  ParallelPVariant=InternalParameters  IdealPVariant=Disabled  IVariant=InternalParameters  DVariant=InternalParameters  IntegratorVariant=Discrete  SatVariant=Enabled  AWVariant=DiscClampingParallel  PCopyVariant=Disabled  TRVariant=Disabled  FdbkBlocksVariant=Forward  IdealPFdbkVariant=Disabled  SatFdbkVariant=Disabled  DerivativeFilterVariant=ForwardEulerFilter  NVariant=InternalParameters  NCopyVariant=Disabled  FilterICVariant=InternalICsFilter  IntegratorICVariant=InternalICs  ExternalResetVariant=Disabled  TRSumVariant=Passthrough  SumFdbkVariant=Disabled  SumVariant=Sum_PID  TsampFilterVariant=InternalTs  TsampNgainVariant=Passthrough  TsampIntegralVariant=Passthrough  ExternalSaturationOutDataTypeStr=Inherit: Same as second input
  Discrete PID Controller2 : slpidlib/PID Controller  Controller=PID  Form=Parallel  TimeDomain=Discrete-time  UseExternalTs=off  SampleTime=-1  IntegratorMethod=Forward Euler  FilterMethod=Forward Euler  ControllerParametersSource=internal  P=k_launch_Mz_kp  I=k_launch_Mz_ki  D=k_launch_Mz_kd  UseFilter=on  N=100  TunerSelectOption=Transfer Function Based (PID Tuner App)  InitialConditionSource=internal  InitialConditionForIntegrator=0  InitialConditionForFilter=0  DifferentiatorICPrevScaledInput=0  ExternalReset=none  TrackingMode=off  Kt=1  LimitOutput=on  SatLimitsSource=internal  UpperSaturationLimit=k_launch_Mz_sat_hi  LowerSaturationLimit=k_launch_Mz_sat_lo  LinearizeAsGain=off  AntiWindupMode=none  Kb=1  POutMin=[]  POutMax=[]  IOutMin=[]  IOutMax=[]  DOutMin=[]  DOutMax=[]  NOutMin=[]  NOutMax=[]  SumOutMin=[]  SumOutMax=[]  SaturationOutMin=[]  SaturationOutMax=[]  PParamMin=[]  PParamMax=[]  IParamMin=[]  IParamMax=[]  DParamMin=[]  DParamMax=[]  NParamMin=[]  NParamMax=[]  KbParamMin=[]  KbParamMax=[]  KtParamMin=[]  KtParamMax=[]  KbOutMin=[]  KbOutMax=[]  KtOutMin=[]  KtOutMax=[]  IntegratorOutMin=[]  IntegratorOutMax=[]  FilterOutMin=[]  FilterOutMax=[]  SumI1OutMin=[]  SumI1OutMax=[]  SumI2OutMin=[]  SumI2OutMax=[]  SumI3OutMin=[]  SumI3OutMax=[]  SumI4OutMin=[]  SumI4OutMax=[]  SumDOutMin=[]  SumDOutMax=[]  DifferentiatorOutMin=[]  DifferentiatorOutMax=[]  FilterDiffOutCoefMin=[]  FilterDiffOutCoefMax=[]  ReciprocalOutMin=[]  ReciprocalOutMax=[]  SumDenOutMin=[]  SumDenOutMax=[]  SumNumOutMin=[]  SumNumOutMax=[]  DivideOutMin=[]  DivideOutMax=[]  UdiffTsProdOutMin=[]  UdiffTsProdOutMax=[]  NTsProdOutMin=[]  NTsProdOutMax=[]  UintegralTsProdOutMin=[]  UintegralTsProdOutMax=[]  UngainTsProdOutMin=[]  UngainTsProdOutMax=[]  IntegratorContinuousStateAttributes=''  IntegratorStateMustResolveToSignalObject=off  IntegratorRTWStateStorageClass=Auto  FilterContinuousStateAttributes=''  FilterStateMustResolveToSignalObject=off  FilterRTWStateStorageClass=Auto  ParallelPVariant=InternalParameters  IdealPVariant=Disabled  IVariant=InternalParameters  DVariant=InternalParameters  IntegratorVariant=Discrete  SatVariant=Enabled  AWVariant=Passthrough  PCopyVariant=Disabled  TRVariant=Disabled  FdbkBlocksVariant=Forward  IdealPFdbkVariant=Disabled  SatFdbkVariant=Disabled  DerivativeFilterVariant=ForwardEulerFilter  NVariant=InternalParameters  NCopyVariant=Disabled  FilterICVariant=InternalICsFilter  IntegratorICVariant=InternalICs  ExternalResetVariant=Disabled  TRSumVariant=Passthrough  SumFdbkVariant=Disabled  SumVariant=Sum_PID  TsampFilterVariant=InternalTs  TsampNgainVariant=Passthrough  TsampIntegralVariant=Passthrough  ExternalSaturationOutDataTypeStr=Inherit: Same as second input
  Gain3 : Gain  Gain=-1
  Gain4 : Gain  Gain=-1
  Gain5 : Gain  Gain=-1
  Mux : Mux  Inputs=3
  Mx : Scope  NumInputPorts=2
  My : Scope  NumInputPorts=2
  Mz : Scope  NumInputPorts=2
  Product{,1..3} (4 alike) : Product
  Selector : Selector  InputPortWidth=12  IndexOptions=Index vector (dialog)  Indices=[10]  OutputSizes=1
  Step1 : Step  Time=k_launch_My_t_launch_begin  SampleTime=0
  Step2 : Step  Time=k_launch_Mz_t_launch_begin  SampleTime=0
  Step3 : Step  Time=k_launch_Mz_t_launch_end  SampleTime=0
  Step4 : Step  Time=k_launch_My_t_launch_end  SampleTime=0
  Step5 : Step  Time=k_launch_Mx_t_launch_begin  SampleTime=0
  Step6 : Step  Time=k_launch_M_t_release  Before=1  After=0  SampleTime=0
  Step7 : Step  Time=k_launch_Mx_t_launch_end  SampleTime=0
  Sum{1..4} (4 alike) : Sum  Inputs=+-
  Terminator{,1..5} (6 alike) : Terminator
  Transfer Fcn : TransferFcn  Denominator=[k_launch_Mx_tau 1]
  Transfer Fcn1 : TransferFcn  Denominator=[k_launch_My_tau 1]
  Transfer Fcn2 : TransferFcn  Denominator=[k_launch_Mz_tau 1]
  Mlaunch : Outport
  wires:
  Transfer Fcn/1 -> Mux/1  "launch_Mx"
  Transfer Fcn2/1 -> Mux/3  "launch_Mz"
  Mux/1 -> Product/2
  Step6/1 -> Product/1
  Product/1 -> Mlaunch/1
  Gain4/1 -> Discrete PID Controller/1
  Gain3/1 -> Discrete PID Controller1/1
  Gain5/1 -> Discrete PID Controller2/1
  Discrete PID Controller2/1 -> Transfer Fcn2/1, Mz/2
  Demux/3 -> Product1/2  "Mz_huck_err"
  Discrete PID Controller/1 -> Transfer Fcn/1, Mx/2
  Discrete PID Controller1/1 -> Transfer Fcn1/1, My/2
  Demux1/3 -> Terminator/1
  Demux/1 -> Terminator1/1
  Demux/2 -> Terminator2/1
  Transfer Fcn1/1 -> Mux/2  "launch_My"
  Sum2/1 -> Product1/1
  Step3/1 -> Sum2/2
  Step2/1 -> Sum2/1
  Product1/1 -> Mz/1, Gain5/1
  Product2/1 -> My/1, Gain3/1
  Product3/1 -> Gain4/1, Mx/1
  Demux1/2 -> Product2/2  "My_huck_err"
  Step1/1 -> Sum1/1
  Step4/1 -> Sum1/2
  Sum1/1 -> Product2/1
  Step7/1 -> Sum3/2
  Step5/1 -> Sum3/1
  Sum3/1 -> Product3/1
  Demux3/3 -> Demux1/1  "X_th"
  Demux3/1 -> Terminator3/1  "X_pos"
  Demux3/4 -> Demux/1  "X_w"
  Demux3/2 -> Terminator4/1  "X_vel"
  err/1 -> Demux3/1
  X/1 -> Selector/1
  Selector/1 -> Sum4/2
  Constant/1 -> Sum4/1
  Demux1/1 -> Product3/2  "Mx_huck_err"
  Sum4/1 -> Terminator5/1  "Mx_huck_err"

== system flatball_hummel_mdl_validation_IC/huck-er/X0-desired ==
  Manual Switch : ManualSwitch  CurrentSetting=0
  X0_15mps_5hz : Constant  Commented=on  Value=[-1 -1 -1.25 15.0 1e-4 1e-4 -0.07 0.21 5.03 -14.94 -1.48 5*2*pi]
  X0_crowther_f2302 : Constant  Value=X0_crowther_f2302
  X0_f2302 : Constant  Commented=on  Value=[-0.90 -0.63 -0.91 13.42 -0.41 0.001 -0.07 0.21 5.03 -14.94 -1.48 3700*pi/180]
  X0_hummel_f2302 : Constant  Value=X0_hummel_f2302
  X0_simple : Constant  Commented=on  Value=[0 0 -1.5 15 0 0 10*pi/180 0 0 0 0 50]
  Out2 : Outport
  wires:
  Manual Switch/1 -> Out2/1
  X0_hummel_f2302/1 -> Manual Switch/2
  X0_crowther_f2302/1 -> Manual Switch/1

== system flatball_hummel_mdl_validation_IC/huck-er/stop ==
  X : Inport
  Compare To Constant : simulink/Logic and Bit Operations/Compare To Constant  relop=>=  const=0  OutDataTypeStr=boolean
  Selector : Selector  InputPortWidth=12  IndexOptions=Index vector (dialog)  Indices=[3]  OutputSizes=1
  Stop Simulation : Stop
  wires:
  Selector/1 -> Compare To Constant/1
  Compare To Constant/1 -> Stop Simulation/1
  X/1 -> Selector/1

== system flatball_hummel_mdl_validation_IC/lab/calc-F ==
  X : Inport
  T_c_N : Inport  Port=2
  alpha : Inport  Port=3
  Fg_N : Constant  Value=[0 0 disc.m*amb.g]'
  Terminator : Terminator
  X-to-vel : MATLAB Function  TreatAsAtomicUnit=on
  aero-coeff : Subsystem
  calc-F : MATLAB Function  TreatAsAtomicUnit=on
  q-inf : Subsystem
  F : Outport
  wires:
  X-to-vel/1(vel) -> calc-F/1(vel)
  X/1 -> q-inf/1(X), X-to-vel/1(X)
  T_c_N/1 -> calc-F/2(T_c_N)
  Fg_N/1 -> calc-F/3(Fg_N)
  calc-F/1(F) -> F/1
  q-inf/1(q-inf-S) -> calc-F/6(q_inf_times_S)
  alpha/1 -> aero-coeff/1(alpha)
  aero-coeff/1(Cl) -> calc-F/4(CLift)
  aero-coeff/2(Cd) -> calc-F/5(CDrag)
  q-inf/2(q-inf-S-d) -> Terminator/1

== system flatball_hummel_mdl_validation_IC/lab/calc-M ==
  X : Inport
  T_c_N : Inport  Port=2
  wD_N_inN : Inport  Port=3
  alpha : Inport  Port=4
  Terminator : Terminator
  X-to-vel : MATLAB Function  TreatAsAtomicUnit=on
  aero-coeff : Subsystem
  calc-M : MATLAB Function  TreatAsAtomicUnit=on
  q-inf : Subsystem
  M : Outport
  wires:
  alpha/1 -> aero-coeff/1(alpha)
  calc-M/1(M) -> M/1
  T_c_N/1 -> calc-M/2(T_c_N)
  X/1 -> X-to-vel/1(X), q-inf/1(X)
  X-to-vel/1(vel) -> calc-M/1(vel)
  q-inf/2(q-inf-S-d) -> calc-M/5(q_inf_times_Sd)
  aero-coeff/1(Cm) -> calc-M/4(CMpitch)
  wD_N_inN/1 -> calc-M/3(wD_N_inN)
  q-inf/1(q-inf-S) -> Terminator/1

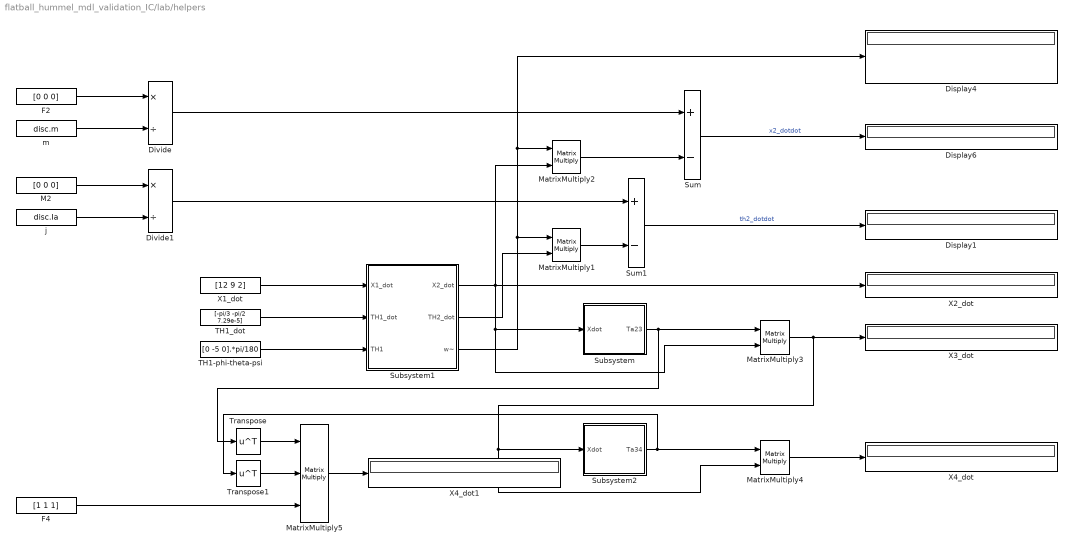
== system flatball_hummel_mdl_validation_IC/lab/helpers ==
  Display1 : Display
  Display4 : Display
  Display6 : Display
  Divide : Product  Inputs=*/
  Divide1 : Product  Inputs=*/
  F2 : Constant  Value=[0 0 0]
  F4 : Constant  Value=[1 1 1]
  M2 : Constant  Value=[0 0 0]
  MatrixMultiply{1..4} (4 alike) : Product  Multiplication=Matrix(*)
  MatrixMultiply5 : Product  Inputs=***  Multiplication=Matrix(*)
  Subsystem : Subsystem
  Subsystem1 : Subsystem
  Subsystem2 : Subsystem
  Sum : Sum  Inputs=+-
  Sum1 : Sum  Inputs=+-
  TH1-phi-theta-psi : Constant  Value=[0 -5 0].*pi/180
  TH1_dot : Constant  Value=[-pi/3 -pi/2 7.29e-5]
  Transpose : Math  Operator=transpose  SaturateOnIntegerOverflow=on
  Transpose1 : Math  Operator=transpose  SaturateOnIntegerOverflow=on
  X1_dot : Constant  Value=[12 9 2]
  X2_dot : Display
  X3_dot : Display
  X4_dot : Display
  X4_dot1 : Display
  j : Constant  Value=disc.Ia
  m : Constant  Value=disc.m
  wires:
  X1_dot/1 -> Subsystem1/1(X1_dot)
  TH1_dot/1 -> Subsystem1/2(TH1_dot)
  TH1-phi-theta-psi/1 -> Subsystem1/3(TH1)
  MatrixMultiply2/1 -> Sum/2
  Subsystem1/3(w~) -> MatrixMultiply1/1, Display4/1, MatrixMultiply2/1
  Subsystem1/1(X2_dot) -> MatrixMultiply2/2, X2_dot/1, MatrixMultiply3/2, Subsystem/1(Xdot)
  F2/1 -> Divide/1
  m/1 -> Divide/2
  Divide/1 -> Sum/1
  Sum/1 -> Display6/1  "x2_dotdot"
  j/1 -> Divide1/2
  M2/1 -> Divide1/1
  Divide1/1 -> Sum1/1
  MatrixMultiply1/1 -> Sum1/2
  Subsystem1/2(TH2_dot) -> MatrixMultiply1/2
  Sum1/1 -> Display1/1  "th2_dotdot"
  Subsystem/1(Ta23) -> Transpose/1, MatrixMultiply3/1
  MatrixMultiply3/1 -> MatrixMultiply4/2, Subsystem2/1(Xdot), X3_dot/1
  Subsystem2/1(Ta34) -> Transpose1/1, MatrixMultiply4/1
  MatrixMultiply4/1 -> X4_dot/1
  Transpose1/1 -> MatrixMultiply5/2
  Transpose/1 -> MatrixMultiply5/1
  F4/1 -> MatrixMultiply5/3
  MatrixMultiply5/1 -> X4_dot1/1

== system flatball_hummel_mdl_validation_IC/lab/rotations ==
  X : Inport
  MatrixMultiply3 : Product  Multiplication=Matrix(*)
  Transpose : Math  Operator=transpose  SaturateOnIntegerOverflow=on
  Transpose1 : Math  Operator=transpose  SaturateOnIntegerOverflow=on
  X-to-T_c_N : MATLAB Function  TreatAsAtomicUnit=on
  X-to-wD_N_inC : MATLAB Function  TreatAsAtomicUnit=on
  T_c_N : Outport
  wD_N : Outport  Port=2
  wires:
  X-to-T_c_N/1(T_c_N) -> Transpose1/1, T_c_N/1
  Transpose1/1 -> MatrixMultiply3/1
  X-to-wD_N_inC/1(wD_N_inC) -> Transpose/1
  Transpose/1 -> MatrixMultiply3/2
  MatrixMultiply3/1 -> wD_N/1
  X/1 -> X-to-wD_N_inC/1(X), X-to-T_c_N/1(X)

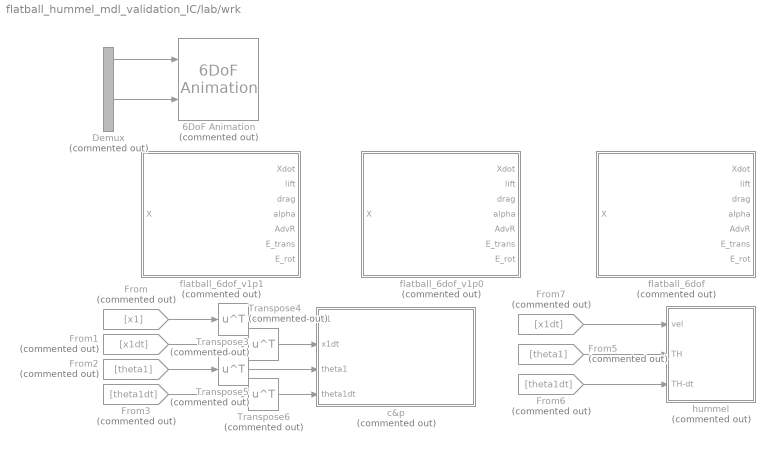
== system flatball_hummel_mdl_validation_IC/lab/wrk ==
  6DoF Animation : aerolibanim/6DoF Animation  Commented=on  u1=[-10 100 -20 100 -10 10]  u2=0.01  u3=5  u4=[1 0 -5]  u5=Fixed position  u6=[100 50 -500]  u7=10  u8=on
  Demux : Demux  Commented=on  Outputs=[3 3 3 3]
  From : From  Commented=on  GotoTag=x1
  From1 : From  Commented=on  GotoTag=x1dt
  From2 : From  Commented=on  GotoTag=theta1
  From3 : From  Commented=on  GotoTag=theta1dt
  From5 : From  Commented=on  GotoTag=theta1
  From6 : From  Commented=on  GotoTag=theta1dt
  From7 : From  Commented=on  GotoTag=x1dt
  Transpose{3..6} (4 alike) : Math  Commented=on  Operator=transpose  SaturateOnIntegerOverflow=on
  c&p : Subsystem  Commented=on
  flatball_6dof : MATLAB Function  Commented=on  TreatAsAtomicUnit=on
  flatball_6dof_v1p0 : MATLAB Function  Commented=on  TreatAsAtomicUnit=on
  flatball_6dof_v1p1 : MATLAB Function  Commented=on  TreatAsAtomicUnit=on
  hummel : Subsystem  Commented=on
  wires:
  From/1 -> Transpose3/1
  From2/1 -> Transpose5/1
  From3/1 -> Transpose6/1
  Demux/3 -> 6DoF Animation/2
  Transpose3/1 -> c&p/1(x1)
  Demux/1 -> 6DoF Animation/1
  From1/1 -> Transpose4/1
  Transpose5/1 -> c&p/3(theta1)
  Transpose4/1 -> c&p/2(x1dt)
  Transpose6/1 -> c&p/4(theta1dt)
  From5/1 -> hummel/2(TH)
  From6/1 -> hummel/3(TH-dt)
  From7/1 -> hummel/1(vel)

== system flatball_hummel_mdl_validation_IC/calc-F/aero-coeff/calc-Cd ==
  alpha : Inport
  Cd0 : Constant  Value=disc.CD0
  Cda : Constant  Value=disc.CDa
  Product : Product
  Square : Math  Operator=square  SaturateOnIntegerOverflow=on
  Sum : Sum  Inputs=+-
  Sum1 : Sum
  alpha0 : Constant  Value=disc.alpha0
  Cd : Outport
  wires:
  Sum1/1 -> Cd/1
  Square/1 -> Product/2
  Product/1 -> Sum1/2
  Cda/1 -> Product/1
  Cd0/1 -> Sum1/1
  Sum/1 -> Square/1
  alpha0/1 -> Sum/2
  alpha/1 -> Sum/1

== system flatball_hummel_mdl_validation_IC/calc-F/aero-coeff/calc-Cl ==
  alpha : Inport
  CL0 : Constant  Value=disc.CL0
  CLa : Constant  Value=disc.CLa
  Product : Product
  Sum1 : Sum
  Cl : Outport
  wires:
  alpha/1 -> Product/2
  CL0/1 -> Sum1/1
  CLa/1 -> Product/1
  Product/1 -> Sum1/2
  Sum1/1 -> Cl/1

== system flatball_hummel_mdl_validation_IC/calc-M/aero-coeff/Subsystem2 ==
  alpha : Inport
  CM0 : Constant  Value=disc.CM0
  CMa : Constant  Value=disc.CMa
  Product : Product
  Sum1 : Sum
  Cm : Outport
  wires:
  Sum1/1 -> Cm/1
  Product/1 -> Sum1/2
  CMa/1 -> Product/1
  CM0/1 -> Sum1/1
  alpha/1 -> Product/2

== system flatball_hummel_mdl_validation_IC/lab/calc-F/aero-coeff ==
  alpha : Inport
  Subsystem : Subsystem
  Subsystem1 : Subsystem
  Cl : Outport
  Cd : Outport  Port=2
  wires:
  alpha/1 -> Subsystem1/1(alpha), Subsystem/1(alpha)
  Subsystem1/1(Cl) -> Cl/1
  Subsystem/1(Cd) -> Cd/1

== system flatball_hummel_mdl_validation_IC/lab/calc-F/q-inf ==
  X : Inport
  Gain : Gain  Gain=0.5
  Product1 : Product  Inputs=3
  Product2 : Product
  S : Constant  Value=disc.A
  Square : Math  Operator=square  SaturateOnIntegerOverflow=on
  X-to-vel : MATLAB Function  TreatAsAtomicUnit=on
  d : Constant  Value=disc.d
  rho : Constant  Value=amb.rho
  vector-norm : MATLAB Function  TreatAsAtomicUnit=on
  q-inf-S : Outport
  q-inf-S-d : Outport  Port=2
  wires:
  Product1/1 -> Gain/1
  rho/1 -> Product1/3
  X/1 -> X-to-vel/1(X)
  vector-norm/1(norm) -> Square/1
  S/1 -> Product1/2
  Square/1 -> Product1/1
  Gain/1 -> Product2/1, q-inf-S/1
  X-to-vel/1(vel) -> vector-norm/1(vec)
  Product2/1 -> q-inf-S-d/1
  d/1 -> Product2/2

== system flatball_hummel_mdl_validation_IC/lab/calc-M/aero-coeff ==
  alpha : Inport
  Subsystem2 : Subsystem
  Cm : Outport
  wires:
  alpha/1 -> Subsystem2/1(alpha)
  Subsystem2/1(Cm) -> Cm/1
